simulink model "zero_crossing_detect"  (Simulink 7.3)
settings: Solver=VariableStepDiscrete  StartTime=0.0  StopTime=10.0  MaxStep=0.01  RelTol=1e-3
settings Model: Creator=sn00632  LastModifiedBy=sn00632
settings SolverCC: MaxConsecutiveZCs=1  ZeroCrossControl=DisableAll

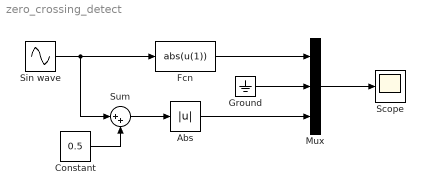
== system zero_crossing_detect ==
  Abs : Abs  OutDataType=fixdt(1, 16)  OutScaling=2^0
  Constant : Constant  Value=0.5  OutDataType=fixdt(1, 16)  OutScaling=2^0
  Fcn : Fcn  Expr=abs(u(1))
  Ground : Ground
  Mux : Mux  Inputs=3
  Scope : Scope
  Sin wave : Sin  Amplitude=1  Bias=0  Frequency=1  Phase=0  Samples=10  SampleTime=0  Offset=0
  Sum : Sum  Inputs=|++  OutDataType=fixdt(1, 16)  OutScaling=2^0
  wires:
  Sin wave/1 -> Fcn/1, Sum/1
  Fcn/1 -> Mux/1
  Mux/1 -> Scope/1
  Ground/1 -> Mux/2
  Abs/1 -> Mux/3
  Constant/1 -> Sum/2
  Sum/1 -> Abs/1
